simulink model "key_ctr_CarSimTest"  (R2016a)
settings: Solver=FixedStepDiscrete  SolverMode=SingleTasking  StartTime=0  StopTime=inf  FixedStep=0.001  RelTol=1e-3  AbsTol=1e-6
PreLoadFcn:
  | PreSettings
InitFcn:
  | set_param(gcs,'StopTime','inf');
settings Model: ExtModeTrigMode=oneshot  ExtModeArmWhenConnect=off  Creator=thomasl  LastModifiedBy=SAIC
settings DataIOCC: SaveFormat=Array  SignalLoggingSaveFormat=ModelDataLogs  SignalLoggingName=sigsOut
settings OptimizationCC: BooleanDataType=off  InitFltsAndDblsToZero=on
settings DebuggingCC: SaveWithParameterizedLinksMsg=none  UnderspecifiedInitializationDetection=Classic  MergeDetectMultiDrivingBlocksExec=none  SignalResolutionControl=TryResolveAllWithWarning  MultiTaskDSMMsg=warning  MultiTaskCondExecSysMsg=none  FcnCallInpInsideContextMsg=UseLocalSettings
settings HardwareCC: ProdBitPerPointer=32  ProdLargestAtomicFloat=None  ProdIntDivRoundTo=Undefined  ProdEndianess=Unspecified  ProdWordSize=32  ProdHWDeviceType=32-bit Generic  TargetBitPerPointer=64  TargetLongLongMode=on  TargetIntDivRoundTo=Zero  TargetEndianess=LittleEndian  TargetWordSize=64  TargetHWDeviceType=MATLAB Host  ProdEqTarget=off
settings ModelReferenceCC: PropagateSignalLabelsOutOfModel=off
settings RTWCC: SystemTargetFile=rtwsfcn.tlc  TemplateMakefile=rtwsfcn_default_tmf
settings CodeAppCC: ForceParamTrailComments=on
settings STFCustomTargetCC: TargetFcnLib=ansi_tfl_tmw.mat  ModelReferenceCompliant=off  MatFileLogging=on  MATLABClassNameForMDSCustomization=Simulink.SoftwareTarget.TargetSpecificTriggerConfigurationBase  SystemTargetFile=rtwsfcn.tlc
settings ConfigComp: CovModelRefEnable=Off

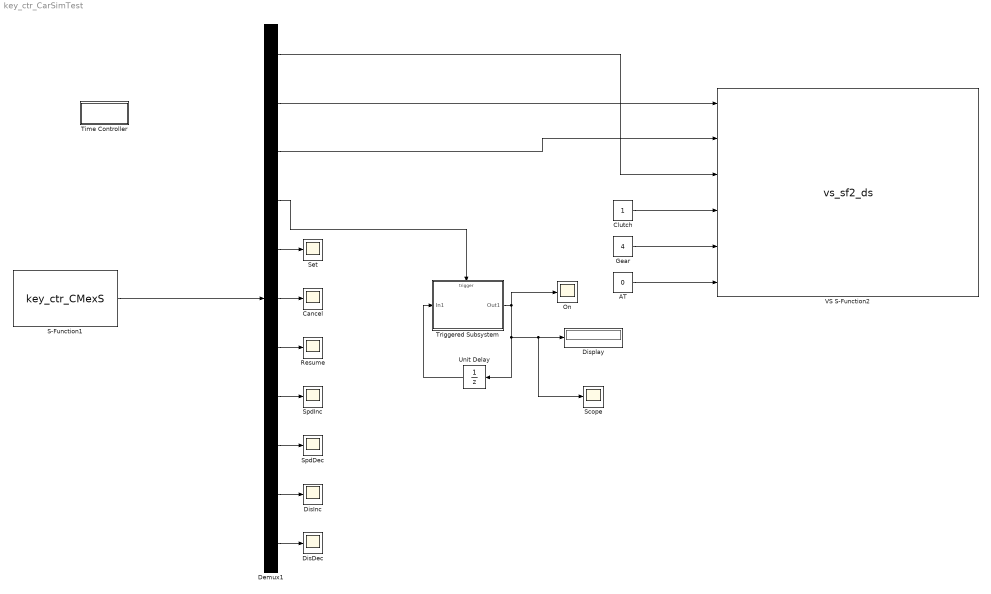
== system key_ctr_CarSimTest ==
  AT : Constant  Value=0
  Cancel : Scope
  Clutch : Constant
  Demux1 : Demux  Outputs=11
  DisDec : Scope
  DisInc : Scope
  Display : Display
  Gear : Constant  Value=4
  On : Scope
  Resume : Scope
  S-Function1 : S-Function  FunctionName=key_ctr_CMexS  SFunctionDeploymentMode=off  EnableBusSupport=off
  Scope : Scope
  Set : Scope
  SpdDec : Scope
  SpdInc : Scope
  Time Controller : Subsystem  mask(CarSim DS){}
      mask help: This Real-Time control block enables the Simulink system running at real time mode.
      mask init:
      | TimeStep=str2num(get_param(gcs,'FixedStep'));
      mask Display: disp('RT Enable');
  Triggered Subsystem : Subsystem  TreatAsAtomicUnit=on
  Unit Delay : UnitDelay  SampleTime=-1
  VS S-Function2 : S-Function  Priority=1  FunctionName=vs_sf2_ds  Parameters='simfile.sim'  SFunctionDeploymentMode=off  EnableBusSupport=off  mask(Vehicle math model library){SIMFILE=simfile.sim}
      mask prompts: SIMFILE "Simfile name:"
      mask help:
      | The vehicle code on this S-Function determine which solver is used for vehicle type that is simulated.
      |
      | Simfile lists the names of the main files that will be read and written by the solver program.
      mask init:
      | set_param(gcb, 'Parameters', ['''',SIMFILE,'''']);
      mask Display: image(imread('car_ds2.bmp'))
  wires:
  Clutch/1 -> VS S-Function2/4
  Gear/1 -> VS S-Function2/5
  AT/1 -> VS S-Function2/6
  S-Function1/1 -> Demux1/1
  Demux1/2 -> VS S-Function2/1
  Demux1/1 -> VS S-Function2/3
  Demux1/3 -> VS S-Function2/2
  Demux1/4 -> Triggered Subsystem/Trigger
  Demux1/5 -> Set/1
  Demux1/6 -> Cancel/1
  Demux1/7 -> Resume/1
  Demux1/8 -> SpdInc/1
  Demux1/9 -> SpdDec/1
  Demux1/10 -> DisInc/1
  Demux1/11 -> DisDec/1
  Triggered Subsystem/1(Out1) -> On/1, Scope/1, Display/1, Unit Delay/1
  Unit Delay/1 -> Triggered Subsystem/1(In1)

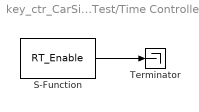
== system key_ctr_CarSimTest/Time Controller ==
  S-Function : S-Function  FunctionName=RT_Enable  Parameters=TimeStep  SFunctionDeploymentMode=off  EnableBusSupport=off
  Terminator : Terminator
  wires:
  S-Function/1 -> Terminator/1

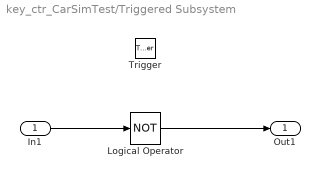
== system key_ctr_CarSimTest/Triggered Subsystem ==
  In1 : Inport
  Trigger : TriggerPort  VariantControl=Variant
  Logical Operator : Logic  Operator=NOT  AllPortsSameDT=off  OutDataTypeStr=boolean
  Out1 : Outport
  wires:
  In1/1 -> Logical Operator/1
  Logical Operator/1 -> Out1/1
